simulink model "and_model_sil"  (R2024a)
settings: Solver=FixedStepDiscrete  StartTime=0.0  StopTime=4  RelTol=1e-3
libraries: spsStairGeneratorLib x2
settings Model: Creator=User  LastModifiedBy=User
settings OptimizationCC: DefaultParameterBehavior=Inlined  EnhancedBackFolding=on  PassReuseOutputArgsAs=Individual arguments  ZeroExternalMemoryAtStartup=off  ZeroInternalMemoryAtStartup=off  OptimizeBlockOrder=speed  DifferentSizesBufferReuse=on  OptimizationCustomize=off  EfficientTunableParamExpr=on
settings DebuggingCC: ParameterTunabilityLossMsg=error
settings SFSimCC: MATLABDynamicMemAlloc=off
settings RTWCC: Description=Embedded Coder  SystemTargetFile=ert.tlc  TemplateMakefile=ert_default_tmf  Toolchain=MinGW64 | gmake (64-bit Windows)
settings CodeAppCC: ForceParamTrailComments=on  IgnoreCustomStorageClasses=off  OperatorAnnotations=on  SimulinkDataObjDesc=on  SFDataObjDesc=on  InsertBlockDesc=on
settings ERTTargetCC: TargetLangStandard=C99 (ISO)  GenerateSampleERTMain=on  InlinedParameterPlacement=NonHierarchical  ERTCustomFileTemplate=example_file_process.tlc
settings ConfigComp: CovEnable=on  CovScope=ReferencedModels  CovIncludeTopModel=off  CovMetricSettings=dcmwe  CovModelRefEnable=filtered

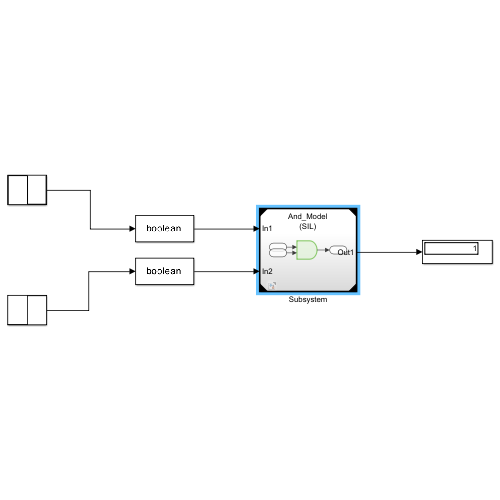
[thumbnail: Simulink's stored preview of the top-level diagram]
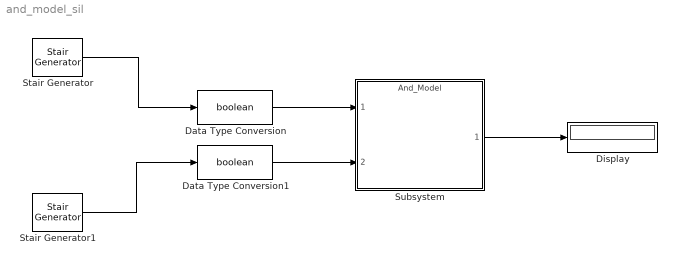
== system and_model_sil ==
  Data Type Conversion : DataTypeConversion  OutDataTypeStr=boolean  SaturateOnIntegerOverflow=off  RndMeth=Floor
  Data Type Conversion1 : DataTypeConversion  OutDataTypeStr=boolean  SaturateOnIntegerOverflow=off  RndMeth=Floor
  Display : Display
  Stair Generator : spsStairGeneratorLib/Stair Generator  t=[0, 1,2,3]  e=[0, 1,0,1]  Ts=1
  Stair Generator1 : spsStairGeneratorLib/Stair Generator  t=[0, 1,2,3]  e=[0,0,1, 1]  Ts=1
  Subsystem : ModelReference  ModelNameDialog=And_Model  SimulationMode=Software-in-the-loop (SIL)  ModelReferenceVersion=1.1
  wires:
  Subsystem/1 -> Display/1
  Stair Generator1/1 -> Data Type Conversion1/1
  Stair Generator/1 -> Data Type Conversion/1
  Data Type Conversion/1 -> Subsystem/1
  Data Type Conversion1/1 -> Subsystem/2
